simulink model "practice1"  (R2020b)
settings: Solver=ode4  StartTime=0.0  StopTime=5  FixedStep=0.001  RelTol=1e-3
settings Model: Creator=yuto  LastModifiedBy=yuto
settings DataIOCC: ReturnWorkspaceOutputs=off

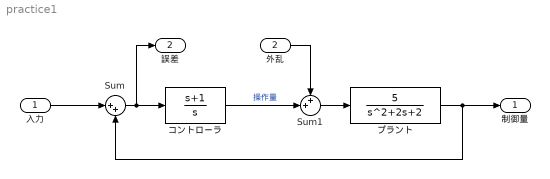
== system practice1 ==
  入力 : Inport
  外乱 : Inport  Port=2
  Sum : Sum  Inputs=|++
  Sum1 : Sum  Inputs=++|
  コントローラ : TransferFcn  Numerator=[1 1]  Denominator=[1 0]
  プラント : TransferFcn  Numerator=[5]  Denominator=[1 2 2]
  制御量 : Outport
  誤差 : Outport  Port=2
  wires:
  Sum/1 -> 誤差/1, コントローラ/1
  プラント/1 -> 制御量/1, Sum/2
  Sum1/1 -> プラント/1
  コントローラ/1 -> Sum1/2  "操作量"
  入力/1 -> Sum/1
  外乱/1 -> Sum1/1
